simulink model "Proyecto_final_sim"  (R2020a)
settings: Solver=VariableStepAuto  StartTime=0.0  StopTime=10.0  RelTol=1e-3
values from neighbouring files (symbols this model uses):
  A = [0 0 1 0 ... (first row only)    [Proyecto_final.m]
  Aob1 = A-L1*C    [Proyecto_final.m]
  Aob_itae = A-L_itae*C    [Proyecto_final.m]
  Aob_lqr = A-L_lqr*C    [Proyecto_final.m]
  Aobcl1 = A-L1*C-B*K1+L1*D*K1    [Proyecto_final.m]
  Aobcl_1 = [Aob1-B*K11+L1*D*K11 -B*Ke ; zeros(1,n) 0]    [Proyecto_final.m]
  Aobcl_1itae = [Aob1_itae-B*K11_itae+L_itae*D*K11_itae -B*Ke_itae ; zeros(1,n) 0]    [Proyecto_final.m]
  Aobcl_1lqr = [Aob_lqr-B*K11_lqr+L_lqr*D*K11_lqr -B*Ke_lqr ; zeros(1,n) 0]    [Proyecto_final.m]
  Aobcl_itae = A-L_itae*C-B*K_itae+L_itae*D*K_itae    [Proyecto_final.m]
  Aobcl_lqr = A-L_lqr*C-B*K_lqr+L_lqr*D*K_lqr    [Proyecto_final.m]
  B = [0;0;(Kg*Ki*n_total)/(Rm*(Jb+m_B*delta_2^2))*(L/d);0]    [Proyecto_final.m]
  Bob1 = [B-L1*D L1]    [Proyecto_final.m]
  Bob_itae = [B-L_itae*D L_itae]    [Proyecto_final.m]
  Bob_lqr = [B-L_lqr*D L_lqr]    [Proyecto_final.m]
  Bobcl1 = [B-L1*D L1]    [Proyecto_final.m]
  Bobcl_1 = [zeros(n,1) L1 ; 1 -1]    [Proyecto_final.m]
  Bobcl_1itae = [zeros(n,1) L_itae ; 1 -1]    [Proyecto_final.m]
  Bobcl_1lqr = [zeros(n,1) L_lqr ; 1 -1]    [Proyecto_final.m]
  Bobcl_itae = [B-L_itae*D L_itae]    [Proyecto_final.m]
  Bobcl_lqr = [B-L_lqr*D L_lqr]    [Proyecto_final.m]
  C = [0 1 0 0]    [Proyecto_final.m]
  Cob1 = eye(4)    [Proyecto_final.m]
  Cob_itae = eye(4)    [Proyecto_final.m]
  Cob_lqr = eye(4)    [Proyecto_final.m]
  Cobcl1 = -K1    [Proyecto_final.m]
  Cobcl_1 = -Kext_1    [Proyecto_final.m]
  Cobcl_1itae = -Kext_itae    [Proyecto_final.m]
  Cobcl_1lqr = -Kext_lqr    [Proyecto_final.m]
  Cobcl_itae = -K_itae    [Proyecto_final.m]
  Cobcl_lqr = -K_lqr    [Proyecto_final.m]
  D = 0    [Proyecto_final.m]
  Dob1 = zeros(rank(A),2)    [Proyecto_final.m]
  Dob_itae = zeros(rank(A),2)    [Proyecto_final.m]
  Dob_lqr = zeros(rank(A),2)    [Proyecto_final.m]
  Dobcl1 = [1 0]    [Proyecto_final.m]
  Dobcl_1 = [0 0]    [Proyecto_final.m]
  Dobcl_1itae = [0 0]    [Proyecto_final.m]
  Dobcl_1lqr = [0 0]    [Proyecto_final.m]
  Dobcl_itae = [1 0]    [Proyecto_final.m]
  Dobcl_lqr = [1 0]    [Proyecto_final.m]
  IP = 1    [Proyecto_final.m]
  K1 = place(A,B,[pole1 pole2 pole3 pole4])    [Proyecto_final.m]
  K_itae = place(A,B,itaepol)    [Proyecto_final.m]
  K_lqr = lqr(A,B,Q,R)    [Proyecto_final.m]
  Kext_1 = place(Aext,Bext,[pole1,pole2,pole3,pole4,pole5])    [Proyecto_final.m]
  Kext_itae = place(Aext,Bext,[pole1_itae,pole2_itae,pole3_itae,pole4_itae,pole5_itae])    [Proyecto_final.m]
  Kext_lqr = lqr(Aext,Bext,Qext,R)    [Proyecto_final.m]
  Kp1 = -inv(((C-D*K1)*inv((A-B*K1))*B-D))    [Proyecto_final.m]
  Kp_itae = -inv(((C-D*K_itae)*inv((A-B*K_itae))*B-D))    [Proyecto_final.m]
  Kp_lqr = -inv(((C-D*K_lqr)*inv((A-B*K_lqr))*B-D))    [Proyecto_final.m]
undefined symbols (not defined in the file or in its folder): rank
settings Model: Creator=Windows_10  LastModifiedBy=Windows_10

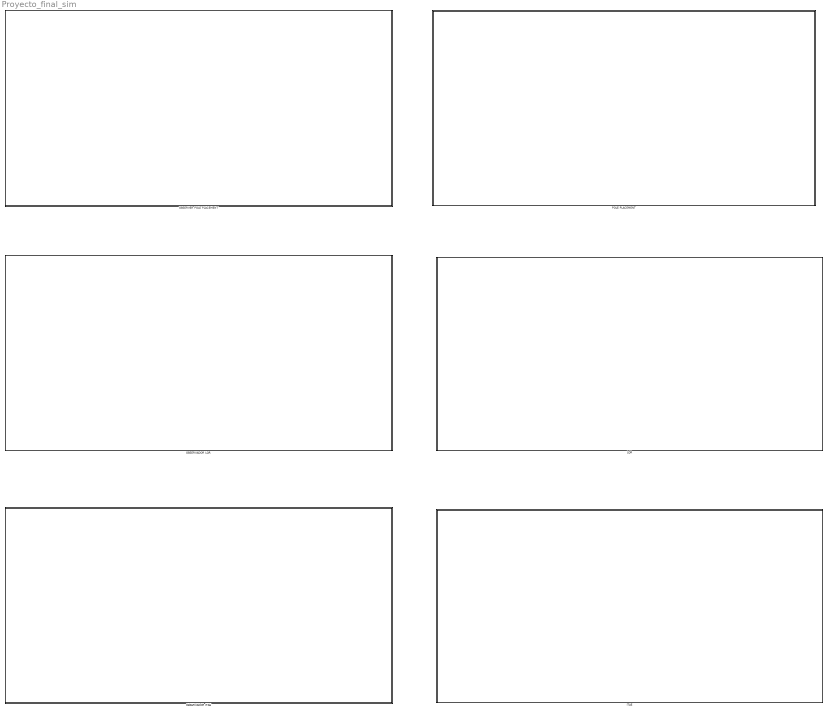
== system Proyecto_final_sim ==
  ITAE : Subsystem
  LQR : Subsystem
  OBSERVADOR ITAE : Subsystem
  OBSERVADOR LQR : Subsystem
  "OBSERVER POLE PLACEMENT " : Subsystem
  POLE PLACEMENT : Subsystem

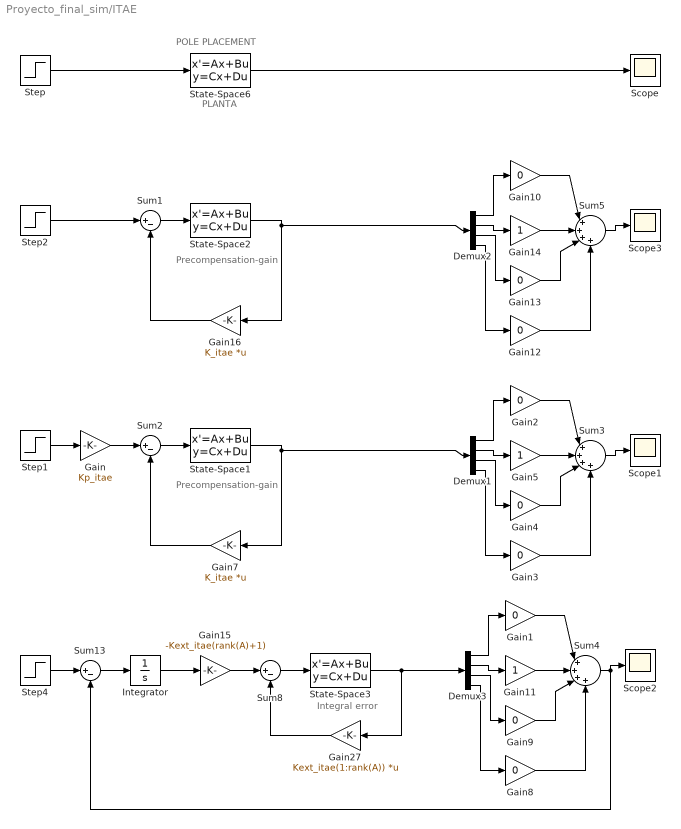
== system Proyecto_final_sim/ITAE ==
  note: POLE PLACEMENT
  note: PLANTA
  note: Precompensation-gain
  note: Precompensation-gain
  note: Integral error
  Demux1 : Demux
  Demux2 : Demux
  Demux3 : Demux
  Gain : Gain  Gain=Kp_itae
  Gain{1..4,8..10,12..13} (9 alike) : Gain  Gain=0
  Gain11 : Gain
  Gain14 : Gain
  Gain15 : Gain  Gain=-Kext_itae(rank(A)+1)
  Gain16 : Gain  Gain=K_itae  Multiplication=Matrix(K*u)
  Gain27 : Gain  Gain=Kext_itae(1:rank(A))  Multiplication=Matrix(K*u)
  Gain5 : Gain
  Gain7 : Gain  Gain=K_itae  Multiplication=Matrix(K*u)
  Integrator : Integrator
  Scope{,1..3} (4 alike) : Scope
  State-Space1 : StateSpace  A=A  B=B  C=eye(rank(A))  D=zeros(rank(A),1)  InitialCondition=0
  State-Space2 : StateSpace  A=A  B=B  C=eye(rank(A))  D=zeros(rank(A),1)  InitialCondition=0
  State-Space3 : StateSpace  A=A*IP  B=B*IP  C=eye(rank(A))  D=zeros(rank(A),1)  InitialCondition=0
  State-Space6 : StateSpace  A=A  B=B  C=eye(rank(A))  D=zeros(rank(A),1)  InitialCondition=0
  Step{,1..2,4} (4 alike) : Step  Time=0  SampleTime=0
  Sum{1..2,8,13} (4 alike) : Sum  Inputs=|+-
  Sum3 : Sum  Inputs=|++++
  Sum4 : Sum  Inputs=|++++
  Sum5 : Sum  Inputs=|++++
  wires:
  State-Space6/1 -> Scope/1
  Sum2/1 -> State-Space1/1
  Step/1 -> State-Space6/1
  Gain/1 -> Sum2/1
  Gain7/1 -> Sum2/2
  Step1/1 -> Gain/1
  Sum3/1 -> Scope1/1
  Gain5/1 -> Sum3/2
  Demux1/1 -> Gain2/1
  Demux1/4 -> Gain3/1
  Gain2/1 -> Sum3/1
  Demux1/3 -> Gain4/1
  Gain4/1 -> Sum3/3
  Demux1/2 -> Gain5/1
  State-Space1/1 -> Demux1/1, Gain7/1
  Gain3/1 -> Sum3/4
  Demux2/3 -> Gain13/1
  Gain10/1 -> Sum5/1
  Demux2/4 -> Gain12/1
  Gain14/1 -> Sum5/2
  Sum5/1 -> Scope3/1
  Demux2/2 -> Gain14/1
  Step2/1 -> Sum1/1
  Gain12/1 -> Sum5/4
  Gain16/1 -> Sum1/2
  State-Space2/1 -> Demux2/1, Gain16/1
  Gain13/1 -> Sum5/3
  Sum1/1 -> State-Space2/1
  Demux2/1 -> Gain10/1
  Gain8/1 -> Sum4/4
  Demux3/3 -> Gain9/1
  Sum8/1 -> State-Space3/1
  Gain1/1 -> Sum4/1
  Gain11/1 -> Sum4/2
  Demux3/2 -> Gain11/1
  Gain9/1 -> Sum4/3
  Demux3/1 -> Gain1/1
  Gain15/1 -> Sum8/1
  Demux3/4 -> Gain8/1
  Sum13/1 -> Integrator/1
  Step4/1 -> Sum13/1
  Gain27/1 -> Sum8/2
  Sum4/1 -> Sum13/2, Scope2/1
  Integrator/1 -> Gain15/1
  State-Space3/1 -> Gain27/1, Demux3/1

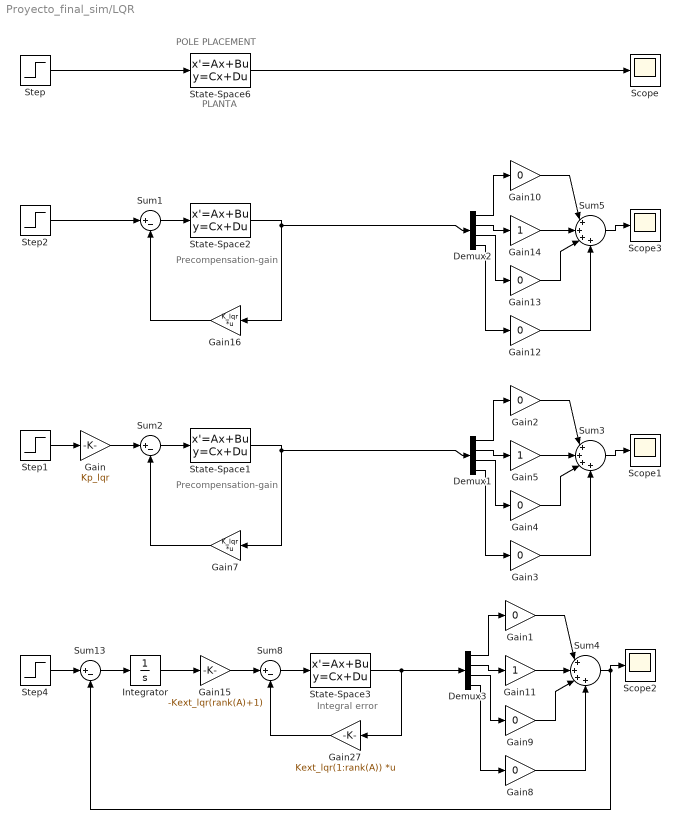
== system Proyecto_final_sim/LQR ==
  note: POLE PLACEMENT
  note: PLANTA
  note: Precompensation-gain
  note: Precompensation-gain
  note: Integral error
  Demux1 : Demux
  Demux2 : Demux
  Demux3 : Demux
  Gain : Gain  Gain=Kp_lqr
  Gain{1..4,8..10,12..13} (9 alike) : Gain  Gain=0
  Gain11 : Gain
  Gain14 : Gain
  Gain15 : Gain  Gain=-Kext_lqr(rank(A)+1)
  Gain16 : Gain  Gain=K_lqr  Multiplication=Matrix(K*u)
  Gain27 : Gain  Gain=Kext_lqr(1:rank(A))  Multiplication=Matrix(K*u)
  Gain5 : Gain
  Gain7 : Gain  Gain=K_lqr  Multiplication=Matrix(K*u)
  Integrator : Integrator
  Scope{,1..3} (4 alike) : Scope
  State-Space1 : StateSpace  A=A  B=B  C=eye(rank(A))  D=zeros(rank(A),1)  InitialCondition=0
  State-Space2 : StateSpace  A=A  B=B  C=eye(rank(A))  D=zeros(rank(A),1)  InitialCondition=0
  State-Space3 : StateSpace  A=A*IP  B=B*IP  C=eye(rank(A))  D=zeros(rank(A),1)  InitialCondition=0
  State-Space6 : StateSpace  A=A  B=B  C=eye(rank(A))  D=zeros(rank(A),1)  InitialCondition=0
  Step{,1..2,4} (4 alike) : Step  Time=0  SampleTime=0
  Sum{1..2,8,13} (4 alike) : Sum  Inputs=|+-
  Sum3 : Sum  Inputs=|++++
  Sum4 : Sum  Inputs=|++++
  Sum5 : Sum  Inputs=|++++
  wires:
  State-Space6/1 -> Scope/1
  Sum2/1 -> State-Space1/1
  Step/1 -> State-Space6/1
  Gain/1 -> Sum2/1
  Gain7/1 -> Sum2/2
  Step1/1 -> Gain/1
  Sum3/1 -> Scope1/1
  Gain5/1 -> Sum3/2
  Demux1/1 -> Gain2/1
  Demux1/4 -> Gain3/1
  Gain2/1 -> Sum3/1
  Demux1/3 -> Gain4/1
  Gain4/1 -> Sum3/3
  Demux1/2 -> Gain5/1
  State-Space1/1 -> Demux1/1, Gain7/1
  Gain3/1 -> Sum3/4
  Demux2/3 -> Gain13/1
  Gain10/1 -> Sum5/1
  Demux2/4 -> Gain12/1
  Gain14/1 -> Sum5/2
  Sum5/1 -> Scope3/1
  Demux2/2 -> Gain14/1
  Step2/1 -> Sum1/1
  Gain12/1 -> Sum5/4
  Gain16/1 -> Sum1/2
  State-Space2/1 -> Demux2/1, Gain16/1
  Gain13/1 -> Sum5/3
  Sum1/1 -> State-Space2/1
  Demux2/1 -> Gain10/1
  Gain8/1 -> Sum4/4
  Demux3/3 -> Gain9/1
  Sum8/1 -> State-Space3/1
  Gain1/1 -> Sum4/1
  Gain11/1 -> Sum4/2
  Demux3/2 -> Gain11/1
  Gain9/1 -> Sum4/3
  Demux3/1 -> Gain1/1
  Gain15/1 -> Sum8/1
  Demux3/4 -> Gain8/1
  Sum13/1 -> Integrator/1
  Step4/1 -> Sum13/1
  Gain27/1 -> Sum8/2
  Sum4/1 -> Sum13/2, Scope2/1
  Integrator/1 -> Gain15/1
  State-Space3/1 -> Gain27/1, Demux3/1

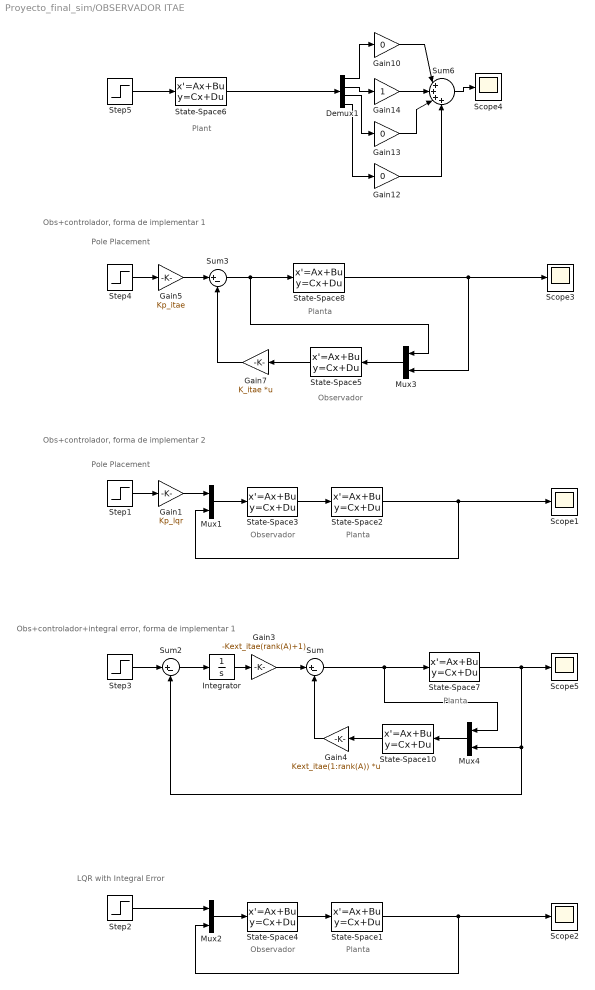
== system Proyecto_final_sim/OBSERVADOR ITAE ==
  note: Planta
  note: Planta
  note: Plant
  note: Observador
  note: Pole Placement
  note: Observador
  note: Pole Placement
  note: Obs+controlador, forma de implementar 1
  note: Obs+controlador, forma de implementar 2
  note: Observador
  note: Planta
  note: LQR with Integral Error
  note: Obs+controlador+integral error, forma de implementar 1
  note: Planta
  Demux1 : Demux
  Gain1 : Gain  Gain=Kp_lqr
  Gain10 : Gain  Gain=0
  Gain12 : Gain  Gain=0
  Gain13 : Gain  Gain=0
  Gain14 : Gain
  Gain3 : Gain  Gain=-Kext_itae(rank(A)+1)
  Gain4 : Gain  Gain=Kext_itae(1:rank(A))  Multiplication=Matrix(K*u)
  Gain5 : Gain  Gain=Kp_itae
  Gain7 : Gain  Gain=K_itae  Multiplication=Matrix(K*u)
  Integrator : Integrator
  Mux{1..4} (4 alike) : Mux  Inputs=2
  Scope{1..5} (5 alike) : Scope
  State-Space{1..2,7..8} (4 alike) : StateSpace  A=A  B=B  C=C  D=D  InitialCondition=0
  State-Space10 : StateSpace  A=Aob_itae  B=Bob_itae  C=Cob_itae  D=Dob_itae  InitialCondition=0
  State-Space3 : StateSpace  A=Aobcl_itae  B=Bobcl_itae  C=Cobcl_itae  D=Dobcl_itae  InitialCondition=0
  State-Space4 : StateSpace  A=Aobcl_1itae  B=Bobcl_1itae  C=Cobcl_1itae  D=Dobcl_1itae  InitialCondition=0
  State-Space5 : StateSpace  A=Aob_itae  B=Bob_itae  C=Cob_itae  D=Dob_itae  InitialCondition=0
  State-Space6 : StateSpace  A=A  B=B  C=eye(rank(A))  D=zeros(rank(A),1)  InitialCondition=0
  Step{1..5} (5 alike) : Step  Time=0  SampleTime=0
  Sum : Sum  Inputs=|+-
  Sum2 : Sum  Inputs=|+-
  Sum3 : Sum  Inputs=|+-
  Sum6 : Sum  Inputs=|++++
  wires:
  Gain7/1 -> Sum3/2
  State-Space2/1 -> Mux1/2, Scope1/1
  Demux1/2 -> Gain14/1
  State-Space3/1 -> State-Space2/1
  Demux1/3 -> Gain13/1
  Gain1/1 -> Mux1/1
  Gain13/1 -> Sum6/3
  Mux1/1 -> State-Space3/1
  State-Space5/1 -> Gain7/1
  Step4/1 -> Gain5/1
  Step5/1 -> State-Space6/1
  Gain5/1 -> Sum3/1
  Mux3/1 -> State-Space5/1
  Sum3/1 -> Mux3/1, State-Space8/1
  State-Space8/1 -> Scope3/1, Mux3/2
  Demux1/1 -> Gain10/1
  State-Space6/1 -> Demux1/1
  Step1/1 -> Gain1/1
  Gain10/1 -> Sum6/1
  Sum6/1 -> Scope4/1
  Gain14/1 -> Sum6/2
  Demux1/4 -> Gain12/1
  Gain12/1 -> Sum6/4
  Mux2/1 -> State-Space4/1
  State-Space1/1 -> Mux2/2, Scope2/1
  State-Space4/1 -> State-Space1/1
  Step2/1 -> Mux2/1
  Integrator/1 -> Gain3/1
  Gain3/1 -> Sum/1
  Step3/1 -> Sum2/1
  Mux4/1 -> State-Space10/1
  State-Space10/1 -> Gain4/1
  Sum2/1 -> Integrator/1
  Sum/1 -> State-Space7/1, Mux4/1
  Gain4/1 -> Sum/2
  State-Space7/1 -> Sum2/2, Mux4/2, Scope5/1

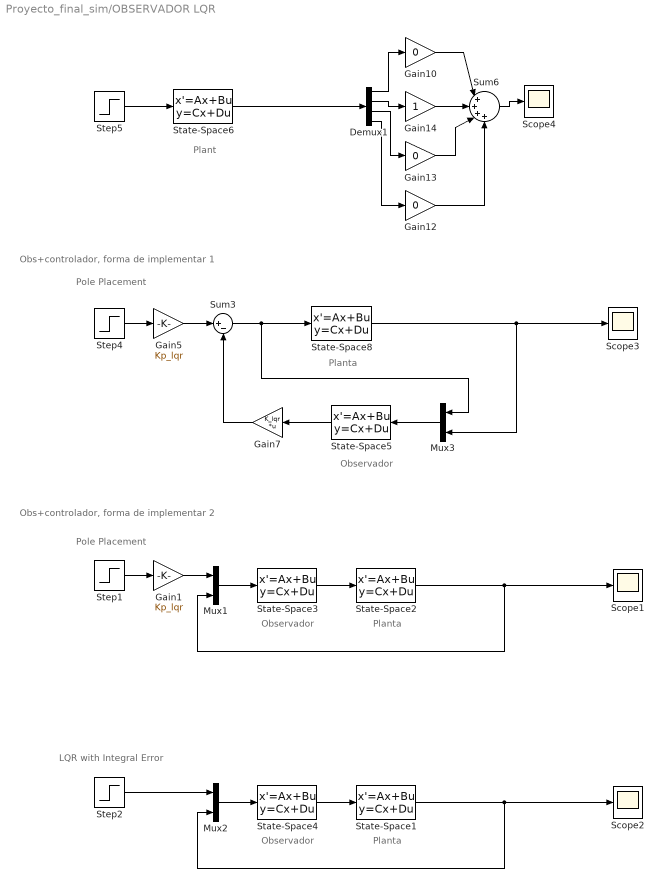
== system Proyecto_final_sim/OBSERVADOR LQR ==
  note: Planta
  note: Planta
  note: Plant
  note: Observador
  note: Pole Placement
  note: Observador
  note: Pole Placement
  note: Obs+controlador, forma de implementar 1
  note: Obs+controlador, forma de implementar 2
  note: Observador
  note: Planta
  note: LQR with Integral Error
  Demux1 : Demux
  Gain1 : Gain  Gain=Kp_lqr
  Gain10 : Gain  Gain=0
  Gain12 : Gain  Gain=0
  Gain13 : Gain  Gain=0
  Gain14 : Gain
  Gain5 : Gain  Gain=Kp_lqr
  Gain7 : Gain  Gain=K_lqr  Multiplication=Matrix(K*u)
  Mux1 : Mux  Inputs=2
  Mux2 : Mux  Inputs=2
  Mux3 : Mux  Inputs=2
  Scope{1..4} (4 alike) : Scope
  State-Space1 : StateSpace  A=A  B=B  C=C  D=D  InitialCondition=0
  State-Space2 : StateSpace  A=A  B=B  C=C  D=D  InitialCondition=0
  State-Space3 : StateSpace  A=Aobcl_lqr  B=Bobcl_lqr  C=Cobcl_lqr  D=Dobcl_lqr  InitialCondition=0
  State-Space4 : StateSpace  A=Aobcl_1lqr  B=Bobcl_1lqr  C=Cobcl_1lqr  D=Dobcl_1lqr  InitialCondition=0
  State-Space5 : StateSpace  A=Aob_lqr  B=Bob_lqr  C=Cob_lqr  D=Dob_lqr  InitialCondition=0
  State-Space6 : StateSpace  A=A  B=B  C=eye(rank(A))  D=zeros(rank(A),1)  InitialCondition=0
  State-Space8 : StateSpace  A=A  B=B  C=C  D=D  InitialCondition=0
  Step{1..2,4..5} (4 alike) : Step  Time=0  SampleTime=0
  Sum3 : Sum  Inputs=|+-
  Sum6 : Sum  Inputs=|++++
  wires:
  Gain7/1 -> Sum3/2
  State-Space2/1 -> Mux1/2, Scope1/1
  Demux1/2 -> Gain14/1
  State-Space3/1 -> State-Space2/1
  Demux1/3 -> Gain13/1
  Gain1/1 -> Mux1/1
  Gain13/1 -> Sum6/3
  Mux1/1 -> State-Space3/1
  State-Space5/1 -> Gain7/1
  Step4/1 -> Gain5/1
  Step5/1 -> State-Space6/1
  Gain5/1 -> Sum3/1
  Mux3/1 -> State-Space5/1
  Sum3/1 -> Mux3/1, State-Space8/1
  State-Space8/1 -> Scope3/1, Mux3/2
  Demux1/1 -> Gain10/1
  State-Space6/1 -> Demux1/1
  Step1/1 -> Gain1/1
  Gain10/1 -> Sum6/1
  Sum6/1 -> Scope4/1
  Gain14/1 -> Sum6/2
  Demux1/4 -> Gain12/1
  Gain12/1 -> Sum6/4
  Mux2/1 -> State-Space4/1
  State-Space1/1 -> Mux2/2, Scope2/1
  State-Space4/1 -> State-Space1/1
  Step2/1 -> Mux2/1

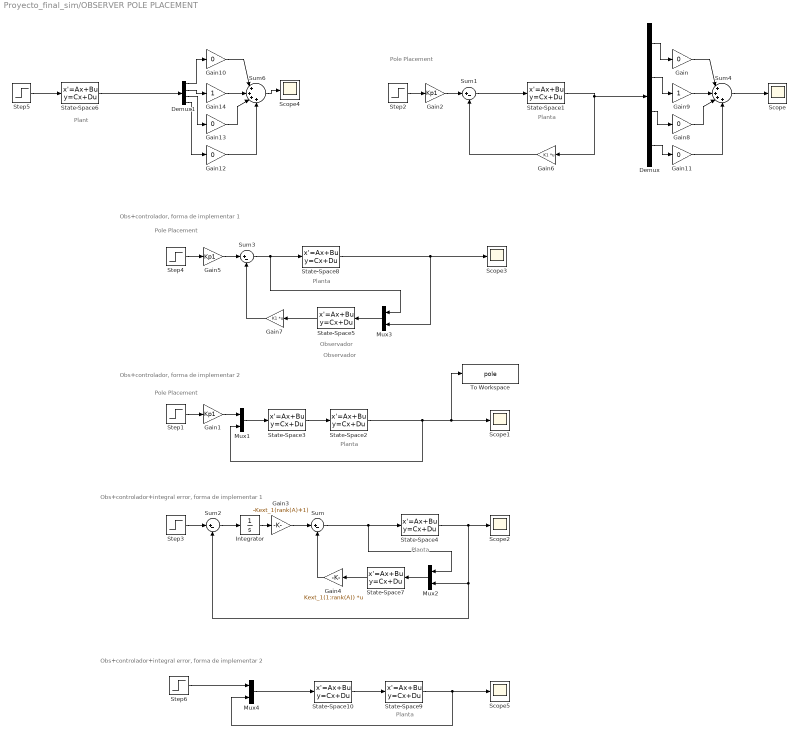
== system Proyecto_final_sim/OBSERVER POLE PLACEMENT  ==
  note: Planta
  note: Planta
  note: Planta
  note: Planta
  note: Planta
  note: Plant
  note: Obs+controlador+integral error, forma de implementar 1
  note: Observador
  note: Pole Placement
  note: Pole Placement
  note: Observador
  note: Pole Placement
  note: Obs+controlador, forma de implementar 1
  note: Obs+controlador, forma de implementar 2
  note: Obs+controlador+integral error, forma de implementar 2
  Demux : Demux
  Demux1 : Demux
  Gain{,8,10..13} (6 alike) : Gain  Gain=0
  Gain1 : Gain  Gain=Kp1
  Gain14 : Gain
  Gain2 : Gain  Gain=Kp1
  Gain3 : Gain  Gain=-Kext_1(rank(A)+1)
  Gain4 : Gain  Gain=Kext_1(1:rank(A))  Multiplication=Matrix(K*u)
  Gain5 : Gain  Gain=Kp1
  Gain6 : Gain  Gain=K1  Multiplication=Matrix(K*u)
  Gain7 : Gain  Gain=K1  Multiplication=Matrix(K*u)
  Gain9 : Gain
  Integrator : Integrator
  Mux{1..4} (4 alike) : Mux  Inputs=2
  Scope{,1..5} (6 alike) : Scope
  State-Space1 : StateSpace  A=A  B=B  C=eye(rank(A))  D=zeros(rank(A),1)  InitialCondition=0
  State-Space10 : StateSpace  A=Aobcl_1  B=Bobcl_1  C=Cobcl_1  D=Dobcl_1  InitialCondition=0
  State-Space{2,4,8..9} (4 alike) : StateSpace  A=A  B=B  C=C  D=D  InitialCondition=0
  State-Space3 : StateSpace  A=Aobcl1  B=Bobcl1  C=Cobcl1  D=Dobcl1  InitialCondition=0
  State-Space5 : StateSpace  A=Aob1  B=Bob1  C=Cob1  D=Dob1  InitialCondition=0
  State-Space6 : StateSpace  A=A  B=B  C=eye(rank(A))  D=zeros(rank(A),1)  InitialCondition=0
  State-Space7 : StateSpace  A=Aob1  B=Bob1  C=Cob1  D=Dob1  InitialCondition=0
  Step{1..6} (6 alike) : Step  Time=0  SampleTime=0
  Sum{,1..3} (4 alike) : Sum  Inputs=|+-
  Sum4 : Sum  Inputs=|++++
  Sum6 : Sum  Inputs=|++++
  To Workspace : ToWorkspace  VariableName=pole  SaveFormat=Timeseries  SampleTime=-1
  wires:
  Gain4/1 -> Sum/2
  Gain7/1 -> Sum3/2
  Gain6/1 -> Sum1/2
  State-Space2/1 -> Mux1/2, To Workspace/1, Scope1/1
  Sum/1 -> State-Space4/1, Mux2/1
  Demux1/2 -> Gain14/1
  State-Space3/1 -> State-Space2/1
  Demux1/3 -> Gain13/1
  Demux/2 -> Gain9/1
  Gain1/1 -> Mux1/1
  Gain13/1 -> Sum6/3
  Step3/1 -> Sum2/1
  Mux1/1 -> State-Space3/1
  State-Space5/1 -> Gain7/1
  Step4/1 -> Gain5/1
  Step5/1 -> State-Space6/1
  Gain5/1 -> Sum3/1
  Sum1/1 -> State-Space1/1
  State-Space4/1 -> Sum2/2, Mux2/2, Scope2/1
  Mux3/1 -> State-Space5/1
  Sum3/1 -> Mux3/1, State-Space8/1
  Gain2/1 -> Sum1/1
  State-Space8/1 -> Scope3/1, Mux3/2
  Mux4/1 -> State-Space10/1
  Demux/1 -> Gain/1
  Mux2/1 -> State-Space7/1
  State-Space7/1 -> Gain4/1
  Step2/1 -> Gain2/1
  Gain/1 -> Sum4/1
  Step6/1 -> Mux4/1
  Demux1/1 -> Gain10/1
  Sum2/1 -> Integrator/1
  State-Space6/1 -> Demux1/1
  Step1/1 -> Gain1/1
  Gain10/1 -> Sum6/1
  Gain3/1 -> Sum/1
  Integrator/1 -> Gain3/1
  State-Space1/1 -> Demux/1, Gain6/1
  State-Space9/1 -> Mux4/2, Scope5/1
  Gain8/1 -> Sum4/3
  Sum6/1 -> Scope4/1
  Gain14/1 -> Sum6/2
  Gain9/1 -> Sum4/2
  Sum4/1 -> Scope/1
  Demux/3 -> Gain8/1
  State-Space10/1 -> State-Space9/1
  Demux/4 -> Gain11/1
  Gain11/1 -> Sum4/4
  Demux1/4 -> Gain12/1
  Gain12/1 -> Sum6/4

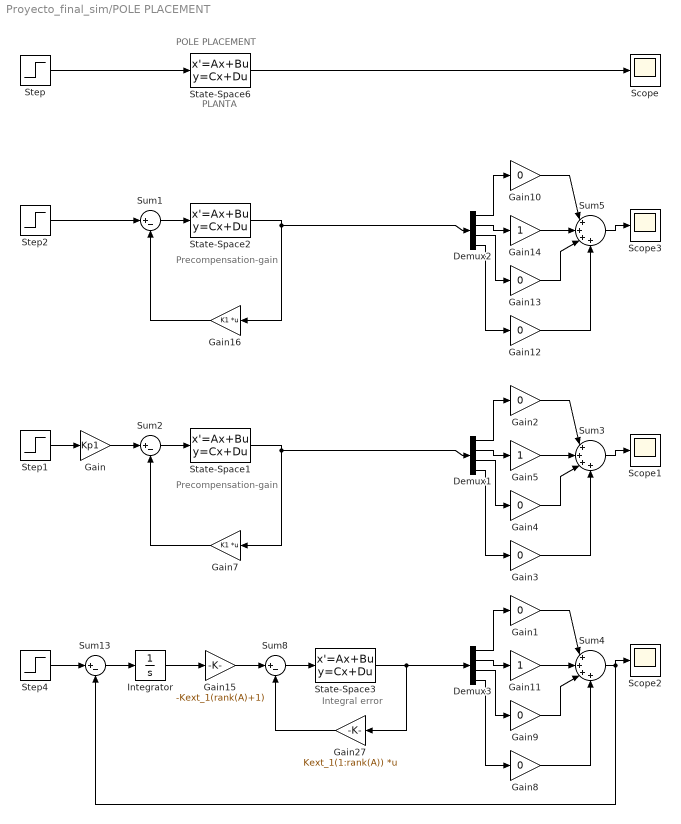
== system Proyecto_final_sim/POLE PLACEMENT ==
  note: POLE PLACEMENT
  note: PLANTA
  note: Precompensation-gain
  note: Integral error
  note: Precompensation-gain
  Demux1 : Demux
  Demux2 : Demux
  Demux3 : Demux
  Gain : Gain  Gain=Kp1
  Gain{1..4,8..10,12..13} (9 alike) : Gain  Gain=0
  Gain11 : Gain
  Gain14 : Gain
  Gain15 : Gain  Gain=-Kext_1(rank(A)+1)
  Gain16 : Gain  Gain=K1  Multiplication=Matrix(K*u)
  Gain27 : Gain  Gain=Kext_1(1:rank(A))  Multiplication=Matrix(K*u)
  Gain5 : Gain
  Gain7 : Gain  Gain=K1  Multiplication=Matrix(K*u)
  Integrator : Integrator
  Scope{,1..3} (4 alike) : Scope
  State-Space1 : StateSpace  A=A*IP  B=B*IP  C=eye(rank(A))  D=zeros(rank(A),1)  InitialCondition=0
  State-Space2 : StateSpace  A=A*IP  B=B  C=eye(rank(A))  D=zeros(rank(A),1)  InitialCondition=0
  State-Space3 : StateSpace  A=A*IP  B=B*IP  C=eye(rank(A))  D=zeros(rank(A),1)  InitialCondition=0
  State-Space6 : StateSpace  A=A  B=B  C=eye(rank(A))  D=zeros(rank(A),1)  InitialCondition=0
  Step{,1..2,4} (4 alike) : Step  Time=0  SampleTime=0
  Sum{1..2,8,13} (4 alike) : Sum  Inputs=|+-
  Sum3 : Sum  Inputs=|++++
  Sum4 : Sum  Inputs=|++++
  Sum5 : Sum  Inputs=|++++
  wires:
  State-Space6/1 -> Scope/1
  Gain27/1 -> Sum8/2
  Sum13/1 -> Integrator/1
  Gain15/1 -> Sum8/1
  Sum2/1 -> State-Space1/1
  Step/1 -> State-Space6/1
  Sum8/1 -> State-Space3/1
  Gain/1 -> Sum2/1
  Gain7/1 -> Sum2/2
  Step4/1 -> Sum13/1
  Step1/1 -> Gain/1
  Integrator/1 -> Gain15/1
  Sum3/1 -> Scope1/1
  Gain5/1 -> Sum3/2
  Demux1/1 -> Gain2/1
  Demux1/4 -> Gain3/1
  Gain2/1 -> Sum3/1
  Demux1/3 -> Gain4/1
  Gain4/1 -> Sum3/3
  Demux1/2 -> Gain5/1
  State-Space1/1 -> Demux1/1, Gain7/1
  Gain3/1 -> Sum3/4
  State-Space3/1 -> Gain27/1, Demux3/1
  Demux3/3 -> Gain9/1
  Demux3/4 -> Gain8/1
  Demux3/1 -> Gain1/1
  Sum4/1 -> Sum13/2, Scope2/1
  Gain8/1 -> Sum4/4
  Gain9/1 -> Sum4/3
  Gain11/1 -> Sum4/2
  Gain1/1 -> Sum4/1
  Demux3/2 -> Gain11/1
  Demux2/3 -> Gain13/1
  Gain10/1 -> Sum5/1
  Demux2/4 -> Gain12/1
  Gain14/1 -> Sum5/2
  Sum5/1 -> Scope3/1
  Demux2/2 -> Gain14/1
  Step2/1 -> Sum1/1
  Gain12/1 -> Sum5/4
  Gain16/1 -> Sum1/2
  State-Space2/1 -> Demux2/1, Gain16/1
  Gain13/1 -> Sum5/3
  Sum1/1 -> State-Space2/1
  Demux2/1 -> Gain10/1
